simulink model "Simulator_6DOF"  (R2017a)
settings: Solver=VariableStepAuto  StartTime=0.0  StopTime=simulation_time  RelTol=1e-3  EnableMultiTasking=on
InitFcn:
  | Parameters_6DOF
values from neighbouring files (symbols this model uses):
  air_density = 1.225    [Parameters_6DOF.m]    (also in parameters.m)
  b = 7    [Parameters_6DOF.m]    (also in parameters.m)
  c = 3    [Parameters_6DOF.m]    (also in parameters.m)
  CD_0_parachute = 0.15    [Parameters_6DOF.m]    (also in parameters.m)
  CD_0_payload = 0.4    [Parameters_6DOF.m]    (also in parameters.m)
  CD_alpha_parachute = 1    [Parameters_6DOF.m]    (also in parameters.m)
  CD_alpha_payload = 2    [Parameters_6DOF.m]    (also in parameters.m)
  CD_dalpha = 0.0001    [Parameters_6DOF.m]    (also in parameters.m)
  CD_ds = 0.3    [Parameters_6DOF.m]    (also in parameters.m)
  CL_0_parachute = 0.4    [Parameters_6DOF.m]    (also in parameters.m)
  CL_alpha_parachute = 2    [Parameters_6DOF.m]    (also in parameters.m)
  Cl_beta = -0.05    [Parameters_6DOF.m]
  CL_dalpha = 0.0001    [Parameters_6DOF.m]    (also in parameters.m)
  Cl_dalpha = 0.0021    [Parameters_6DOF.m]    (also in parameters.m)
  CL_ds = 0.21    [Parameters_6DOF.m]    (also in parameters.m)
  Cl_p = -0.1    [Parameters_6DOF.m]    (also in parameters.m)
  Cm_0 = 0.018    [Parameters_6DOF.m]    (also in parameters.m)
  Cm_alpha = -0.2    [Parameters_6DOF.m]    (also in parameters.m)
  Cm_q = -2    [Parameters_6DOF.m]    (also in parameters.m)
  Cn_dalpha = 0.004    [Parameters_6DOF.m]    (also in parameters.m)
  Cn_r = -0.07    [Parameters_6DOF.m]    (also in parameters.m)
  degToRad = pi/180    (= 0.0174532925199)    [Parameters_6DOF.m]    (also in parameters.m)
  gravity = 9.81    [Parameters_6DOF.m]    (also in parameters.m)
  inertia_tensor = [2.5  0   0 ... (first row only)    [Parameters_6DOF.m]    (also in parameters.m)
  inertia_tensor_inv = inertia_tensor\eye(3)    [Parameters_6DOF.m]    (also in parameters.m)
  initial_position = [0 0 -1000]'    [Main.m]    (also in parameters.m)
  mass = mass_parachute + mass_body    (= 148)    [Parameters_6DOF.m]    (also in parameters.m)
  mass_matrix = diag([mass mass mass])    [Parameters_6DOF.m]    (also in parameters.m)
  mass_matrix_inv = mass_matrix\eye(3)    [Parameters_6DOF.m]    (also in parameters.m)
  S_parachute = 21    [Parameters_6DOF.m]    (also in parameters.m)
  S_payload = 0.5    [Parameters_6DOF.m]    (also in parameters.m)
  X_gb = [0, 0, 0.5]'    [Parameters_6DOF.m]    (also in parameters.m)
  X_gp = [0, 0, -7.5]'    [Parameters_6DOF.m]    (also in parameters.m)
undefined symbols (not defined in the file or in its folder): Cl_r, Cn_beta, Cn_p, Cy_beta, magnitude
libraries: sharedutil x2, aerolibutil x2, aerolibasang x2
settings Model: Creator=Mattia  LastModifiedBy=extra
settings DataIOCC: SaveFormat=Array
settings OptimizationCC: LifeSpan=inf
settings DebuggingCC: SFUnexpectedBacktrackingDiag=warning  SFNoUnconditionalDefaultTransitionDiag=warning  SFExecutionAtInitializationDiag=none
settings GRTTargetCC: TargetLangStandard=C89/C90 (ANSI)  GeneratePreprocessorConditionals=Disable all
settings ConfigComp: CovMetricSettings=dw  CovHtmlReporting=on  CovSaveCumulativeToWorkspaceVar=on  CovSaveSingleToWorkspaceVar=on  CovExternalEMLEnable=off

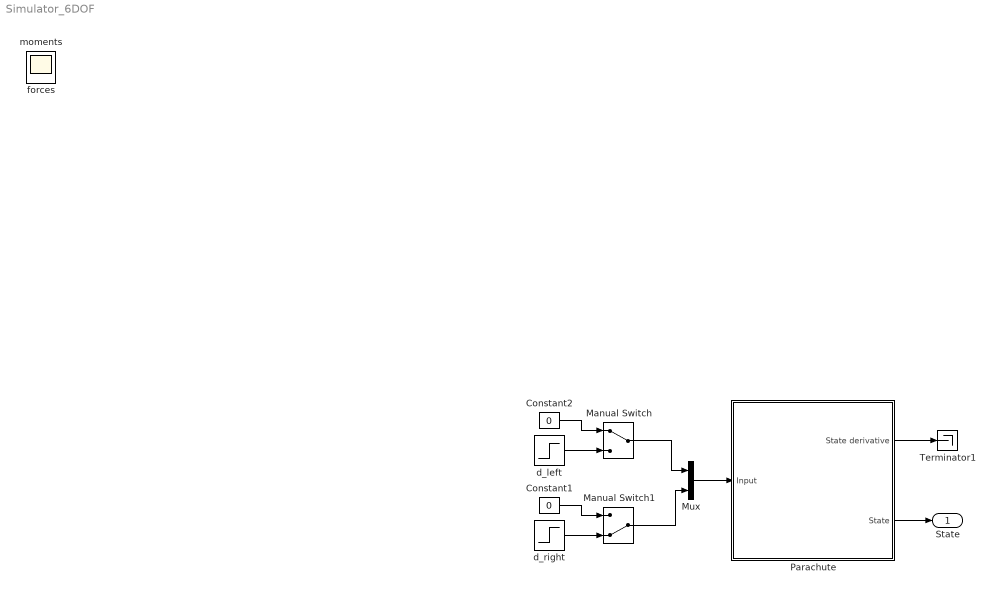
== system Simulator_6DOF ==
  Constant1 : Constant  Value=0
  Constant2 : Constant  Value=0
  Manual Switch : ManualSwitch
  Manual Switch1 : ManualSwitch  CurrentSetting=0
  Mux : Mux  Inputs=2
  Parachute : Subsystem
      mask Display:
      | image(imread('common/rogallo.jpg'))
      | port_label('input',1,'u')
      | port_label('output',1,'Xdot')
      | port_label('output',2,'X')
  Terminator1 : Terminator
  d_left : Step  Time=20  After=20 * degToRad  SampleTime=0
  d_right : Step  Time=50  After=20 * degToRad  SampleTime=0
  State : Outport
  forces : Scope
  moments : Scope
  wires:
  Parachute/1(State derivative) -> Terminator1/1
  Parachute/2(State) -> State/1
  Mux/1 -> Parachute/1(Input)
  Manual Switch/1 -> Mux/1
  d_left/1 -> Manual Switch/2
  Manual Switch1/1 -> Mux/2
  Constant1/1 -> Manual Switch1/1
  d_right/1 -> Manual Switch1/2
  Constant2/1 -> Manual Switch/1

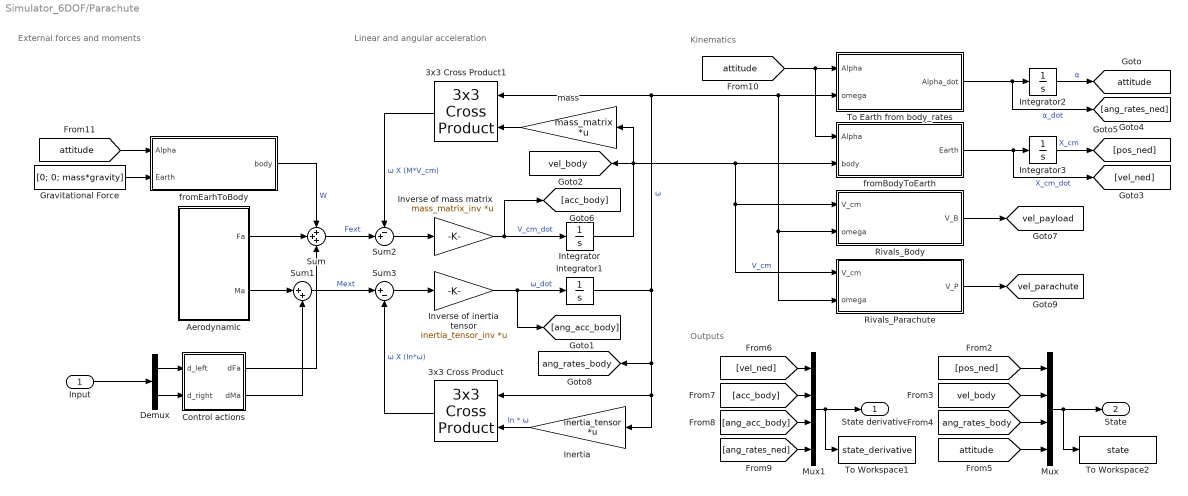
== system Simulator_6DOF/Parachute ==
  note: Outputs
  note: Kinematics
  note: Linear and angular acceleration
  note: External forces and moments
  Input : Inport
  3x3 Cross Product : sharedutil/3x3 Cross Product
  3x3 Cross Product1 : sharedutil/3x3 Cross Product
  Aerodynamic : Subsystem
  Control actions : Subsystem
  Demux : Demux  Outputs=2
  Gravitational Force : Constant  Value=[0; 0; mass*gravity]
  Inertia : Gain  Gain=inertia_tensor  Multiplication=Matrix(K*u)
  Integrator : Integrator  InitialCondition=[0; 0; 0.1]
  Integrator1 : Integrator  InitialCondition=[0; 0; 0]
  Integrator2 : Integrator  InitialCondition=[0; 0; 0]
  Integrator3 : Integrator  InitialCondition=initial_position
  Inverse of inertia tensor : Gain  Gain=inertia_tensor_inv  Multiplication=Matrix(K*u)
  Inverse of mass matrix : Gain  Gain=mass_matrix_inv  Multiplication=Matrix(K*u)
  Mux : Mux
  Mux1 : Mux
  Rivals_Body : MATLAB Function  TreatAsAtomicUnit=on
  Rivals_Parachute : MATLAB Function  TreatAsAtomicUnit=on
  Sum : Sum  Inputs=+++
  Sum1 : Sum  Inputs=|++
  Sum2 : Sum  Inputs=-+|
  Sum3 : Sum  Inputs=|+-
  To Earth from body_rates : MATLAB Function  TreatAsAtomicUnit=on
  To Workspace1 : ToWorkspace  VariableName=state_derivative  SaveFormat=Timeseries  SampleTime=0.01
  To Workspace2 : ToWorkspace  VariableName=state  SaveFormat=Timeseries  SampleTime=0.01
  fromBodyToEarth : MATLAB Function  TreatAsAtomicUnit=on
  fromEarhToBody : MATLAB Function  TreatAsAtomicUnit=on
  mass : Gain  Gain=mass_matrix  Multiplication=Matrix(K*u)
  State derivative : Outport
  State : Outport  Port=2
  tag scope: ang_rates_body=global, attitude=global, vel_body=global, vel_parachute=global, vel_payload=global
  wires:
  To Earth from body_rates/1(Alpha_dot) -> [ang_rates_ned], Integrator2/1  "α_dot"
  [pos_ned] -> Mux/1
  3x3 Cross Product/1 -> Sum3/2  "ω X (In*ω)"
  [acc_body] -> Mux1/2
  Mux/1 -> To Workspace2/1, State/1
  Mux1/1 -> To Workspace1/1, State derivative/1
  [vel_body] -> Mux/2
  [attitude] -> Mux/4
  [ang_rates_body] -> Mux/3
  [ang_rates_ned] -> Mux1/4
  [ang_acc_body] -> Mux1/3
  [vel_ned] -> Mux1/1
  Inverse of mass matrix/1 -> Integrator/1, [acc_body]  "V_cm_dot"
  Integrator/1 -> mass/1, [vel_body], Rivals_Parachute/1(V_cm), Rivals_Body/1(V_cm), fromBodyToEarth/2(body)  "V_cm"
  [attitude] -> fromBodyToEarth/1(Alpha), To Earth from body_rates/1(Alpha)
  Integrator1/1 -> Rivals_Parachute/2(omega), Rivals_Body/2(omega), To Earth from body_rates/2(omega), 3x3 Cross Product1/1, Inertia/1, 3x3 Cross Product/1, [ang_rates_body]  "ω"
  Sum3/1 -> Inverse of inertia tensor/1
  Sum2/1 -> Inverse of mass matrix/1
  mass/1 -> 3x3 Cross Product1/2
  Sum/1 -> Sum2/2  "Fext"
  Inverse of inertia tensor/1 -> [ang_acc_body], Integrator1/1  "ω_dot"
  3x3 Cross Product1/1 -> Sum2/1  "ω X (M*V_cm)"
  Integrator2/1 -> [attitude]  "α"
  Integrator3/1 -> [pos_ned]  "X_cm"
  Inertia/1 -> 3x3 Cross Product/2  "In * ω"
  fromBodyToEarth/1(Earth) -> [vel_ned], Integrator3/1  "X_cm_dot"
  fromEarhToBody/1(body) -> Sum/1  "W"
  Gravitational Force/1 -> fromEarhToBody/2(Earth)
  [attitude] -> fromEarhToBody/1(Alpha)
  Rivals_Body/1(V_B) -> [vel_payload]
  Rivals_Parachute/1(V_P) -> [vel_parachute]
  Aerodynamic/1(Fa) -> Sum/2
  Sum1/1 -> Sum3/1  "Mext"
  Aerodynamic/2(Ma) -> Sum1/1
  Control actions/1(dFa) -> Sum/3
  Control actions/2(dMa) -> Sum1/2
  Demux/1 -> Control actions/1(d_left)
  Demux/2 -> Control actions/2(d_right)
  Input/1 -> Demux/1

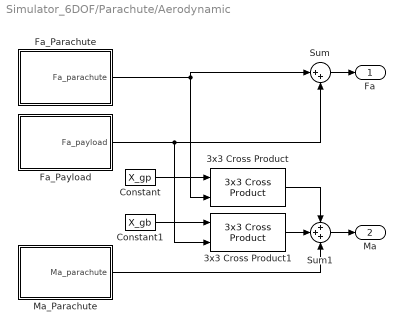
== system Simulator_6DOF/Parachute/Aerodynamic ==
  3x3 Cross Product : aerolibutil/3x3 Cross Product
      settings: SourceProductName=Aerospace Blockset  SourceProductBaseCode=AE
  3x3 Cross Product1 : aerolibutil/3x3 Cross Product
      settings: SourceProductName=Aerospace Blockset  SourceProductBaseCode=AE
  Constant : Constant  Value=X_gp
  Constant1 : Constant  Value=X_gb
  Fa_Parachute : Subsystem
  Fa_Payload : Subsystem
  Ma_Parachute : Subsystem
  Sum : Sum  Inputs=|++
  Sum1 : Sum  Inputs=+++
  Fa : Outport
  Ma : Outport  Port=2
  wires:
  Fa_Payload/1(Fa_payload) -> 3x3 Cross Product1/2, Sum/2
  Sum/1 -> Fa/1
  Fa_Parachute/1(Fa_parachute) -> Sum/1, 3x3 Cross Product/2
  Sum1/1 -> Ma/1
  3x3 Cross Product/1 -> Sum1/1
  Ma_Parachute/1(Ma_parachute) -> Sum1/3
  3x3 Cross Product1/1 -> Sum1/2
  Constant1/1 -> 3x3 Cross Product1/1
  Constant/1 -> 3x3 Cross Product/1

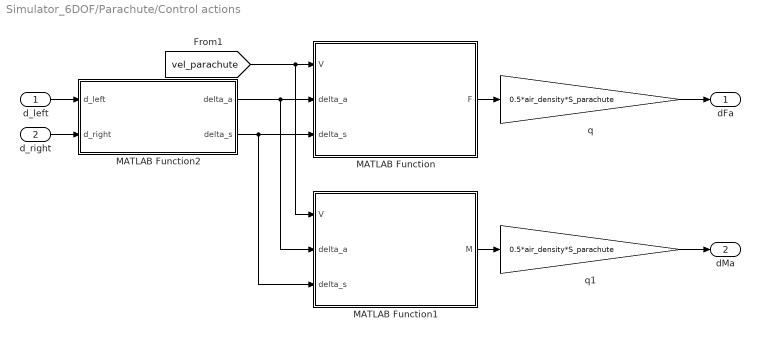
== system Simulator_6DOF/Parachute/Control actions ==
  d_left : Inport
  d_right : Inport  Port=2
  MATLAB Function : MATLAB Function  TreatAsAtomicUnit=on
  MATLAB Function1 : MATLAB Function  TreatAsAtomicUnit=on
  MATLAB Function2 : MATLAB Function  TreatAsAtomicUnit=on
  q : Gain  Gain=0.5*air_density*S_parachute
  q1 : Gain  Gain=0.5*air_density*S_parachute
  dFa : Outport
  dMa : Outport  Port=2
  wires:
  MATLAB Function/1(F) -> q/1
  [vel_parachute] -> MATLAB Function1/1(V), MATLAB Function/1(V)
  q/1 -> dFa/1
  MATLAB Function1/1(M) -> q1/1
  q1/1 -> dMa/1
  d_right/1 -> MATLAB Function2/2(d_right)
  d_left/1 -> MATLAB Function2/1(d_left)
  MATLAB Function2/1(delta_a) -> MATLAB Function1/2(delta_a), MATLAB Function/2(delta_a)
  MATLAB Function2/2(delta_s) -> MATLAB Function1/3(delta_s), MATLAB Function/3(delta_s)

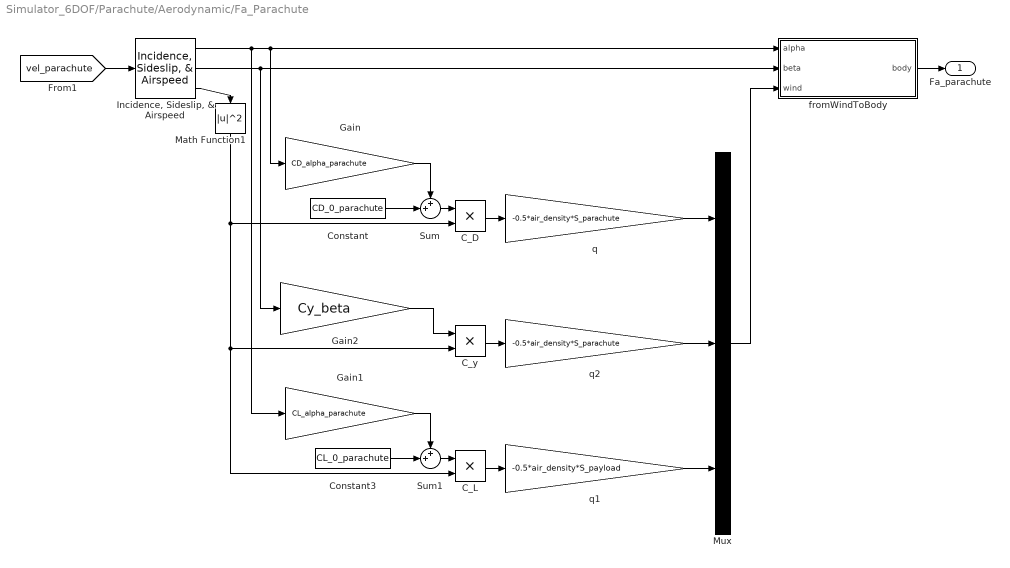
== system Simulator_6DOF/Parachute/Aerodynamic/Fa_Parachute ==
  C_D : Product
  C_L : Product
  C_y : Product
  Constant : Constant  Value=CD_0_parachute
  Constant3 : Constant  Value=CL_0_parachute
  Gain : Gain  Gain=CD_alpha_parachute
  Gain1 : Gain  Gain=CL_alpha_parachute
  Gain2 : Gain  Gain=Cy_beta
  "Incidence, Sideslip, & Airspeed" : aerolibasang/Incidence, Sideslip, & Airspeed
      settings: SourceProductName=Aerospace Blockset
  Math Function1 : Math  Operator=magnitude^2  SaturateOnIntegerOverflow=on
  Mux : Mux  Inputs=3
  Sum : Sum  Inputs=++|
  Sum1 : Sum  Inputs=++|
  fromWindToBody : MATLAB Function  TreatAsAtomicUnit=on
  q : Gain  Gain=-0.5*air_density*S_parachute
  q1 : Gain  Gain=-0.5*air_density*S_payload
  q2 : Gain  Gain=-0.5*air_density*S_parachute
  Fa_parachute : Outport
  wires:
  Math Function1/1 -> C_L/2, C_y/2, C_D/2
  "Incidence, Sideslip, & Airspeed"/1 -> Gain1/1, Gain/1, fromWindToBody/1(alpha)
  Constant/1 -> Sum/2
  Gain/1 -> Sum/1
  Sum/1 -> C_D/1
  "Incidence, Sideslip, & Airspeed"/3 -> Math Function1/1
  C_D/1 -> q/1
  [vel_parachute] -> "Incidence, Sideslip, & Airspeed"/1
  Constant3/1 -> Sum1/2
  Gain1/1 -> Sum1/1
  Sum1/1 -> C_L/1
  q/1 -> Mux/1
  C_L/1 -> q1/1
  q1/1 -> Mux/3
  fromWindToBody/1(body) -> Fa_parachute/1
  Mux/1 -> fromWindToBody/3(wind)
  "Incidence, Sideslip, & Airspeed"/2 -> Gain2/1, fromWindToBody/2(beta)
  C_y/1 -> q2/1
  q2/1 -> Mux/2
  Gain2/1 -> C_y/1

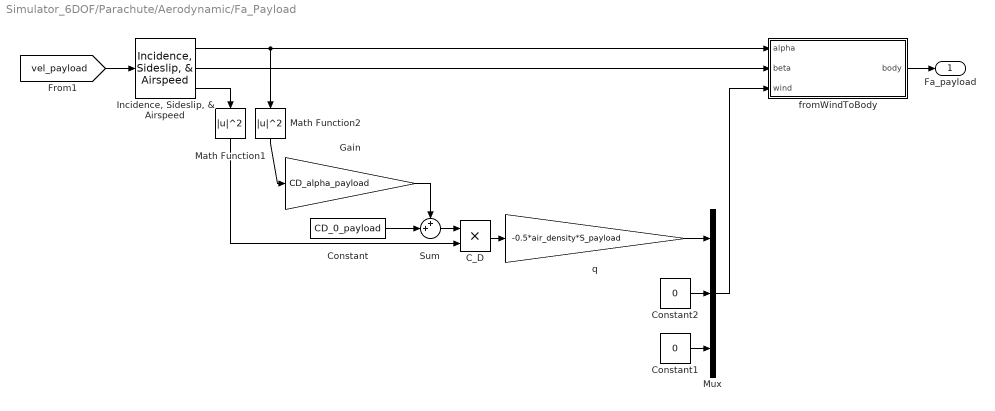
== system Simulator_6DOF/Parachute/Aerodynamic/Fa_Payload ==
  C_D : Product
  Constant : Constant  Value=CD_0_payload
  Constant1 : Constant  Value=0
  Constant2 : Constant  Value=0
  Gain : Gain  Gain=CD_alpha_payload
  "Incidence, Sideslip, & Airspeed" : aerolibasang/Incidence, Sideslip, & Airspeed
      settings: SourceProductName=Aerospace Blockset
  Math Function1 : Math  Operator=magnitude^2  SaturateOnIntegerOverflow=on
  Math Function2 : Math  Operator=magnitude^2  SaturateOnIntegerOverflow=on
  Mux : Mux  Inputs=3
  Sum : Sum  Inputs=++|
  fromWindToBody : MATLAB Function  TreatAsAtomicUnit=on
  q : Gain  Gain=-0.5*air_density*S_payload
  Fa_payload : Outport
  wires:
  Constant2/1 -> Mux/2
  Math Function1/1 -> C_D/2
  Math Function2/1 -> Gain/1
  Constant/1 -> Sum/2
  Gain/1 -> Sum/1
  Sum/1 -> C_D/1
  fromWindToBody/1(body) -> Fa_payload/1
  Constant1/1 -> Mux/3
  C_D/1 -> q/1
  q/1 -> Mux/1
  "Incidence, Sideslip, & Airspeed"/3 -> Math Function1/1
  "Incidence, Sideslip, & Airspeed"/1 -> Math Function2/1, fromWindToBody/1(alpha)
  Mux/1 -> fromWindToBody/3(wind)
  "Incidence, Sideslip, & Airspeed"/2 -> fromWindToBody/2(beta)
  [vel_payload] -> "Incidence, Sideslip, & Airspeed"/1

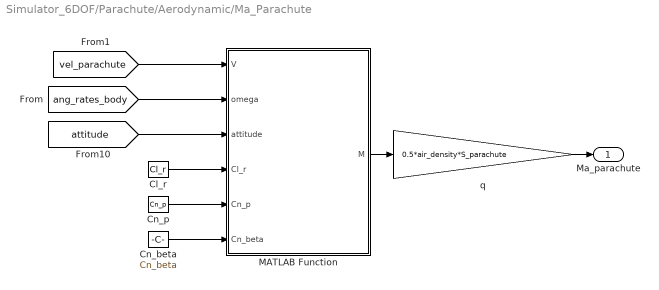
== system Simulator_6DOF/Parachute/Aerodynamic/Ma_Parachute ==
  Cl_r : Constant  Value=Cl_r
  Cn_beta : Constant  Value=Cn_beta
  Cn_p : Constant  Value=Cn_p
  MATLAB Function : MATLAB Function  TreatAsAtomicUnit=on
  q : Gain  Gain=0.5*air_density*S_parachute
  Ma_parachute : Outport
  wires:
  q/1 -> Ma_parachute/1
  MATLAB Function/1(M) -> q/1
  [vel_parachute] -> MATLAB Function/1(V)
  [ang_rates_body] -> MATLAB Function/2(omega)
  [attitude] -> MATLAB Function/3(attitude)
  Cl_r/1 -> MATLAB Function/4(Cl_r)
  Cn_beta/1 -> MATLAB Function/6(Cn_beta)
  Cn_p/1 -> MATLAB Function/5(Cn_p)

== matlab function Simulator_6DOF/Parachute/fromEarhToBody ==
  data: Alpha input; body output; Earth input
 function body = fromEarhToBody(Alpha, Earth)
%#codegen
phi = Alpha(1);
theta = Alpha(2);
psi = Alpha(3);

rotationMatrix = getEarthToBodyMatrix( phi, theta, psi );

body = rotationMatrix * Earth;

== matlab function Simulator_6DOF/Parachute/fromBodyToEarth ==
  data: Alpha input; Earth output; body input
 function Earth = fromBodyToEarth(Alpha, body)
%#codegen
phi = Alpha(1);
theta = Alpha(2);
psi = Alpha(3);

rotationMatrix = getEarthToBodyMatrix( phi, theta, psi )';

Earth = rotationMatrix * body;

== matlab function Simulator_6DOF/Parachute/To Earth from body_rates ==
  data: Alpha input; omega input; Alpha_dot output
 function Alpha_dot = Einv(Alpha, omega)
%#codegen
phi = Alpha(1);
theta = Alpha(2);

Sphi = sin(phi);
Cphi = cos(phi);
Ctheta = cos(theta);
Ttheta = tan(theta);

Einv = [1   Sphi*Ttheta    Cphi*Ttheta ;
        0       Cphi          -Sphi    ;
        0   Sphi/Ctheta    Cphi/Ctheta];

Alpha_dot = Einv * omega;

== matlab function Simulator_6DOF/Parachute/Rivals_Body ==
  data: V_cm input; V_B output; omega input; X_gb parameter
 function V_B = Rivals(V_cm, omega, X_gb)
%#codegen
Omega_cross = getSkew( omega );

V_B = V_cm + Omega_cross * X_gb;

== matlab function Simulator_6DOF/Parachute/Rivals_Parachute ==
  data: V_cm input; V_P output; omega input; X_gp parameter
 function V_P = Rivals(V_cm, omega, X_gp)
%#codegen
Omega_cross = getSkew( omega );

V_P = V_cm + Omega_cross * X_gp;

== matlab function Simulator_6DOF/Parachute/Aerodynamic/Ma_Parachute/MATLAB Function ==
  data: V input; M output; omega input; attitude input; Cl_p parameter; Cm_q parameter; Cn_r parameter; Cl_beta parameter; Cm_0 parameter; Cm_alpha parameter; Cl_r input; Cn_p input; Cn_beta input; b parameter; c parameter
function M = Aero_moments(V, omega, attitude, Cl_p, Cm_q, Cn_r, Cl_beta, Cm_0, Cm_alpha, Cl_r, Cn_p, Cn_beta, b, c) %#ok<INUSL>
alpha_p = atan2(V(3), V(1));
V_abs = sqrt(V(1)^2 + V(2)^2 + V(3)^2);
beta_p=asin(V(2)/V_abs);
% Ahmed: this is the equation to find "Beta" sideslip angle

M = V_abs^2 * [ Cl_p * b^2 * omega(1) / (2 * V_abs ) + Cl_r * b^2 * omega(3) / (2 * V_abs ) + Cl_beta * b * beta_p ;
                Cm_q * c^2 * omega(2) / (2 * V_abs ) + Cm_0 * c + Cm_alpha * c * alpha_p    ;
                Cn_r * b^2 * omega(3) / (2 * V_abs ) + Cn_p * b^2 * omega(1) / (2 * V_abs ) + Cn_beta * b * beta_p];

== matlab function Simulator_6DOF/Parachute/Control actions/MATLAB Function ==
  data: V input; F output; delta_a input; delta_s input; CL_dalpha parameter; CD_dalpha parameter; CL_ds parameter; CD_ds parameter
function F = Control_Forces(V, delta_a, delta_s, CL_dalpha, CD_dalpha , CL_ds, CD_ds)
V_abs = sqrt(V(1)^2 + V(2)^2 + V(3)^2);

S_F = V_abs * [ ( CL_dalpha * V(3) - CD_dalpha * V(1)) * sign(delta_a), ( CL_ds * V(3) - CD_ds * V(1))  ;
                                   - CD_dalpha * V(2)  * sign(delta_a),                - CD_ds * V(2)   ;
                (-CL_dalpha * V(1) - CD_dalpha * V(3)) * sign(delta_a), (-CL_ds * V(1) - CD_ds * V(3)) ];

F = S_F * [ delta_a  ;
            delta_s ];

== matlab function Simulator_6DOF/Parachute/Control actions/MATLAB Function1 ==
  data: V input; M output; delta_a input; delta_s input; Cl_dalpha parameter; Cn_dalpha parameter; b parameter; t parameter
function M = Control_Moments(V, delta_a, delta_s, Cl_dalpha, Cn_dalpha, b, t)
V_abs = sqrt(V(1)^2 + V(2)^2 + V(3)^2);

S_M = V_abs^2 * [ Cl_dalpha * b / t, 0 ;
                                  0, 0 ;
                  Cn_dalpha * b / t, 0];

M = S_M * [ delta_a  ;
            delta_s ];

== matlab function Simulator_6DOF/Parachute/Control actions/MATLAB Function2 ==
  data: d_left input; delta_a output; delta_s output; d_right input
function [delta_a, delta_s] = Control_Actions( d_left, d_right )
delta_a = d_left - d_right;
delta_s = mean([d_left, d_right]);

== matlab function Simulator_6DOF/Parachute/Aerodynamic/Fa_Parachute/fromWindToBody ==
  data: alpha input; beta input; body output; wind input
function body = fromWindToBody(alpha, beta, wind)
%#codegen

rotationMatrix = getWindToBodyMatrix( alpha, beta );

body = rotationMatrix * wind;

== matlab function Simulator_6DOF/Parachute/Aerodynamic/Fa_Payload/fromWindToBody ==
  data: alpha input; beta input; body output; wind input
function body = fromWindToBody(alpha, beta, wind)
%#codegen

rotationMatrix = getWindToBodyMatrix( alpha, beta );

body = rotationMatrix * wind;
